simulink model "fan_predictive_maintenance"  (R2024a)
settings: Solver=ode23t  StartTime=0.0  StopTime=30  RelTol=1e-4  AbsTol=1e-4
libraries: fl_lib x13, nesl_utility x5, ee_lib x1, simulink x1
settings Model: Creator=kzlee  LastModifiedBy=kzlee

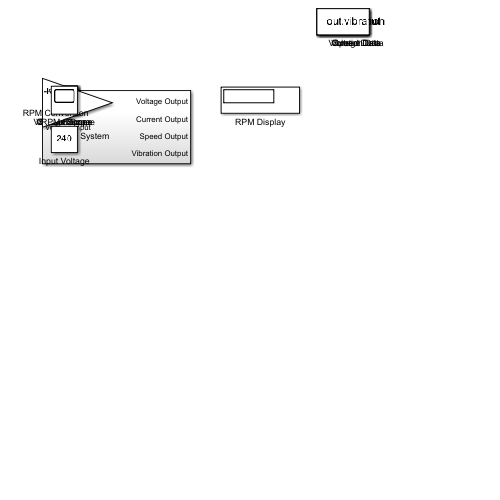
[thumbnail: Simulink's stored preview of the top-level diagram]
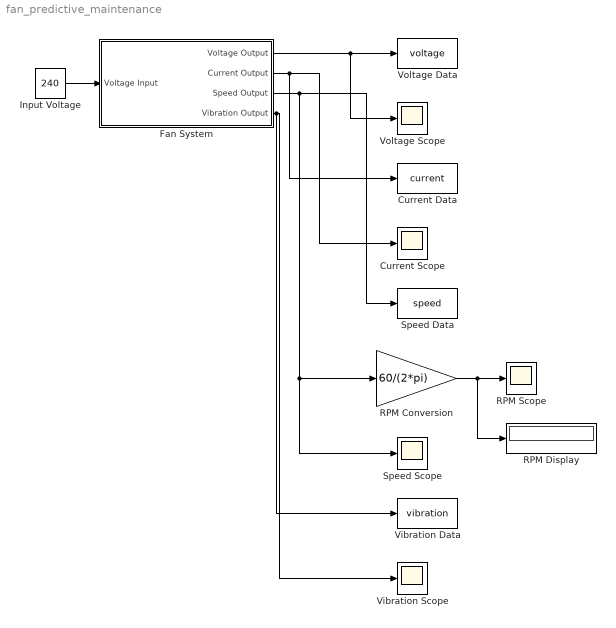
== system fan_predictive_maintenance ==
  Current Data : ToWorkspace  VariableName=current  SaveFormat=Timeseries  SampleTime=-1
  Current Scope : Scope
  Fan System : Subsystem
  Input Voltage : Constant  Value=240
  RPM Conversion : Gain  Gain=60/(2*pi)
  RPM Display : Display
  RPM Scope : Scope
  Speed Data : ToWorkspace  VariableName=speed  SaveFormat=Timeseries  SampleTime=-1
  Speed Scope : Scope
  Vibration Data : ToWorkspace  VariableName=vibration  SaveFormat=Timeseries  SampleTime=-1
  Vibration Scope : Scope
  Voltage Data : ToWorkspace  VariableName=voltage  SaveFormat=Timeseries  SampleTime=-1
  Voltage Scope : Scope
  wires:
  Input Voltage/1 -> Fan System/1(Voltage Input)
  Fan System/3(Speed Output) -> Speed Scope/1, RPM Conversion/1, Speed Data/1
  Fan System/2(Current Output) -> Current Data/1, Current Scope/1
  Fan System/1(Voltage Output) -> Voltage Data/1, Voltage Scope/1
  Fan System/4(Vibration Output) -> Vibration Scope/1, Vibration Data/1
  RPM Conversion/1 -> RPM Display/1, RPM Scope/1

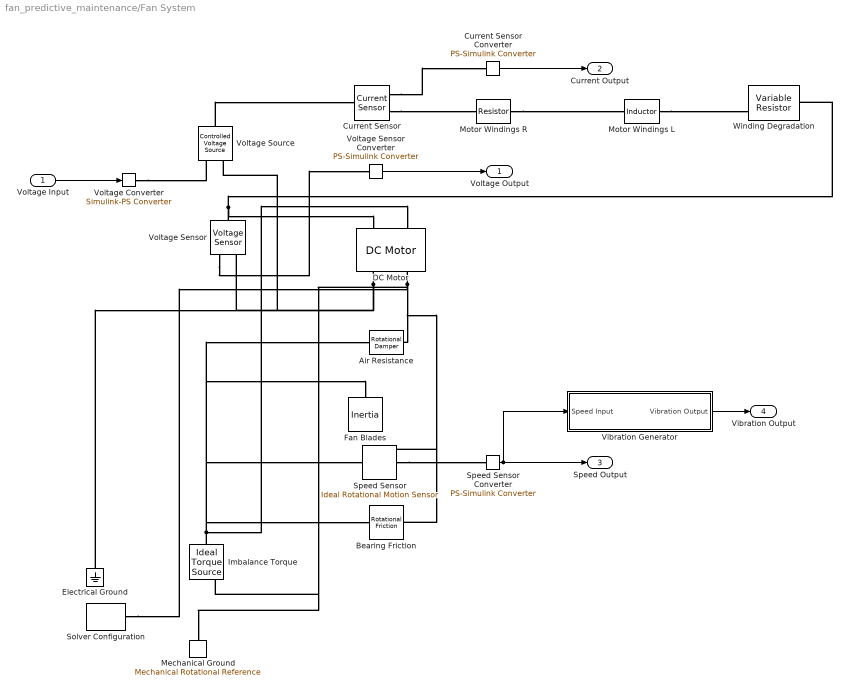
== system fan_predictive_maintenance/Fan System ==
  Voltage Input : Inport
  Air Resistance : fl_lib/Mechanical/Rotational Elements/Rotational Damper  D=0.0045612 N*m*s/rad  w_specify=off  w_priority=None  w=0 rad/s  w_nominal_specify=off  w_nominal_value=1  w_nominal_unit=rad/s  t_specify=off  t_priority=None  t=0 N*m  t_nominal_specify=off  t_nominal_value=1  t_nominal_unit=N*m
  Bearing Friction : fl_lib/Mechanical/Rotational Elements/Rotational Friction  brkwy_trq=25 N*m  brkwy_vel=0.1 rad/s  Col_trq=20 N*m  visc_coef=0.1 N*m*s/rad  w_specify=off  w_priority=None  w=0 rad/s  w_nominal_specify=off  w_nominal_value=1  w_nominal_unit=rad/s  t_specify=off  t_priority=None  t=0 N*m  t_nominal_specify=off  t_nominal_value=1  t_nominal_unit=N*m
  Current Sensor : fl_lib/Electrical/Electrical Sensors/Current Sensor
  Current Sensor Converter : nesl_utility/PS-Simulink Converter  PhysicalDomain=network_engine_domain  SubClassName=ps_output  LeftPortType=input  RightPortType=output  PseudoPeriodic=off  Frequencies=[]  VectorFormat=inherit  Unit=inherit  AffineConversion=off
  DC Motor : ee_lib/Electromechanical/Brushed Motors/DC Motor  field_option=ee.enum.field_option.pm  Rf=100 Ohm  Lf=1 H  Laf=0.15 H  If0=0 A  parameterization=ee.enum.dcparam_option.circuit_param  Ra=1 Ohm  La=0.001 H  emf_or_torque=ee.enum.emf_or_torque.kv  Kv=0.16667 V/rpm  Ki=6.876e-4 N*m/A  T_stall=0.24e-3 N*m  w_max=19100 rpm  w_rated=15000 rpm  P_rated=0.08 W  V_rated=1.5 V  lam_param=ee.enum.lam_param.damping  i_noload=0 A  V_i_noload=1.5 V  J=0.01 cm^2*g  lam=0 N*m*s/rad  speed0=0 rpm  enable_fault_armature=simscape.enum.onoff.off  rev_faulted=1 / 3  G_faulted_armature=1e-5 S  fault_trigger_armature=ee.enum.faults.faultTrigger.temporal  t_fault_armature=1 s  max_permissible_current_armature=inf A  t_fail_on_current_armature=1 s  enable_fault_field=simscape.enum.onoff.off  G_faulted_field=1e-5 S  fault_trigger_field=ee.enum.faults.faultTrigger.temporal  t_fault_field=1 s  max_permissible_current_field=inf A  t_fail_on_current_field=1 s  fault_action=simscape.enum.assert.action.none  alpha=3.93e-3 1/K  Tmeas=25 degC  thermal_mass=100 J/K  initial_temperature=25 degC
  Electrical Ground : fl_lib/Electrical/Electrical Elements/Electrical Reference
  Fan Blades : fl_lib/Mechanical/Rotational Elements/Inertia  inertia=0.001 kg*m^2  num_ports=foundation.enum.numPorts2.one  w_specify=off  w_priority=High  w=0 rad/s  w_nominal_specify=off  w_nominal_value=1  w_nominal_unit=rad/s  t_specify=off  t_priority=None  t=0 N*m  t_nominal_specify=off  t_nominal_value=1  t_nominal_unit=N*m
  Imbalance Torque : fl_lib/Mechanical/Mechanical Sources/Ideal Torque Source
  Mechanical Ground : fl_lib/Mechanical/Rotational Elements/Mechanical Rotational Reference
  Motor Windings L : fl_lib/Electrical/Electrical Elements/Inductor  l=0.001 H  r=0 Ohm  g=1e-9 1/Ohm  i_specify=off  i_priority=None  i=0 A  i_nominal_specify=off  i_nominal_value=1  i_nominal_unit=A  v_specify=off  v_priority=None  v=0 V  v_nominal_specify=off  v_nominal_value=1  v_nominal_unit=V  i_L_specify=off  i_L_priority=High  i_L=0 A  i_L_nominal_specify=off  i_L_nominal_value=1  i_L_nominal_unit=A
  Motor Windings R : fl_lib/Electrical/Electrical Elements/Resistor  R=0.5 Ohm  i_specify=off  i_priority=None  i=0 A  i_nominal_specify=off  i_nominal_value=1  i_nominal_unit=A  v_specify=off  v_priority=None  v=0 V  v_nominal_specify=off  v_nominal_value=1  v_nominal_unit=V
  Solver Configuration : nesl_utility/Solver Configuration  PhysicalDomain=network_engine_domain  SubClassName=solver  LeftPortType=input  RightPortType=generic  Tones=[]  Harmonics=[]  SimulateNoise=off  Profile=off  UseLocalSampling=off  EnableSwitchedLinearOptims=on  FrequencyDomain=off  UseCCode=off  RelTol=0.001  AbsTol=0.001  MinStep=1e-09  ToWorkspace=off  RevertToSquareIcSolve=off  NumHomotopyIterations=100  PhasorMode=off  PhasorModeNumHarmonics=1  ConsistencySolver=NEWTON_XTOL_AFTER_FTOL  IndexReductionMethod=DerivativeReplacement  DoDC=off  ResidualTolerance=1e-09  ConsistencyTolSource=GLOBAL  ConsistencyAbsTol=0.001  ConsistencyRelTol=0.001  ConsistencyTolFactor=0.001  UseLocalSolver=off  LocalSolverChoice=NE_BACKWARD_EULER_ADVANCER  ResolveIndetEquations=on  FunctionEvalNumThread=1  LocalSolverSampleTime=0.001  DoFixedCost=off  MaxNonlinIter=3  MaxModeIter=2  ComputeImpulses=off  ImpulseIterations=2  LinearAlgebra=auto  LinearAlgebraNumThread=0  EquationFormulation=NE_TIME_EF  DelaysMemoryBudget=1024  AutomaticFiltering=on  FilteringTimeConstant=0.001  PartitionStorageMethod=AS_NEEDED  PartitionMemoryBudget=1024  PartitionMethod=ROBUST  MultibodyUseLocalSolver=off  MultibodyLocalSolverChoice=ODE1  MultibodyLocalSolverSampleTime=0.001
  Speed Sensor : fl_lib/Mechanical/Mechanical Sensors/Ideal Rotational Motion Sensor  reference=foundation.enum.MeasurementReference.difference  acceleration_port=false  velocity_port=true  position_port=true  wrap_angle=false  offset=0 rad
  Speed Sensor Converter : nesl_utility/PS-Simulink Converter  PhysicalDomain=network_engine_domain  SubClassName=ps_output  LeftPortType=input  RightPortType=output  PseudoPeriodic=off  Frequencies=[]  VectorFormat=inherit  Unit=inherit  AffineConversion=off
  Vibration Generator : Subsystem
  Voltage Converter : nesl_utility/Simulink-PS Converter  PhysicalDomain=network_engine_domain  SubClassName=ps_input  LeftPortType=input  RightPortType=output  PseudoPeriodic=off  Frequencies=[]  NoiseDistribution=none  NoiseParameters=[]  Unit=1  AffineConversion=off  FilteringAndDerivatives=provide  SimscapeFilterOrder=1  InputFilterTimeConstant=0.001  UdotUserProvided=0
  Voltage Sensor : fl_lib/Electrical/Electrical Sensors/Voltage Sensor
  Voltage Sensor Converter : nesl_utility/PS-Simulink Converter  PhysicalDomain=network_engine_domain  SubClassName=ps_output  LeftPortType=input  RightPortType=output  PseudoPeriodic=off  Frequencies=[]  VectorFormat=inherit  Unit=inherit  AffineConversion=off
  Voltage Source : fl_lib/Electrical/Electrical Sources/Controlled Voltage Source
  Winding Degradation : fl_lib/Electrical/Electrical Elements/Variable Resistor  Rmin=0.1 Ohm  thermalEnable=false  thermal_mass=1 J/K  i_specify=off  i_priority=None  i=0 A  i_nominal_specify=off  i_nominal_value=1  i_nominal_unit=A  v_specify=off  v_priority=None  v=0 V  v_nominal_specify=off  v_nominal_value=1  v_nominal_unit=V  T_specify=off  T_priority=None  T=300 K  T_nominal_specify=off  T_nominal_value=1  T_nominal_unit=K
  Voltage Output : Outport
  Current Output : Outport  Port=2
  Speed Output : Outport  Port=3
  Vibration Output : Outport  Port=4
  wires:
  Voltage Input/1 -> Voltage Converter/1
  Speed Sensor Converter/1 -> Vibration Generator/1(Speed Input), Speed Output/1
  Voltage Sensor Converter/1 -> Voltage Output/1
  Current Sensor Converter/1 -> Current Output/1
  Vibration Generator/1(Vibration Output) -> Vibration Output/1
  connections:
  Voltage Converter/RConn1 -- Voltage Source/RConn1
  Voltage Sensor/LConn1 -- DC Motor/LConn1 -- Winding Degradation/RConn1
  Current Sensor/RConn1 -- Current Sensor Converter/LConn1
  Voltage Sensor/RConn1 -- Voltage Sensor Converter/LConn1
  Current Sensor/RConn2 -- Motor Windings R/LConn1
  Electrical Ground/LConn1 -- Voltage Source/RConn2 -- Voltage Sensor/RConn2 -- DC Motor/RConn1
  Voltage Source/LConn1 -- Current Sensor/LConn1
  Solver Configuration/RConn1 -- Imbalance Torque/RConn2 -- Bearing Friction/RConn1 -- Speed Sensor/RConn1 -- Air Resistance/RConn1 -- Mechanical Ground/LConn1 -- DC Motor/RConn2
  Imbalance Torque/LConn1 -- Air Resistance/LConn1 -- DC Motor/LConn2 -- Speed Sensor/LConn1 -- Bearing Friction/LConn1 -- Fan Blades/LConn1
  Speed Sensor/RConn2 -- Speed Sensor Converter/LConn1
  Motor Windings R/RConn1 -- Motor Windings L/LConn1
  Motor Windings L/RConn1 -- Winding Degradation/LConn2

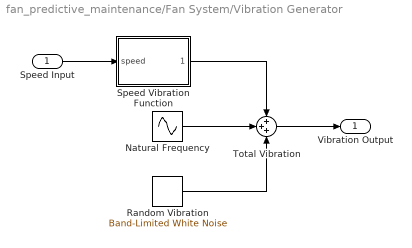
== system fan_predictive_maintenance/Fan System/Vibration Generator ==
  Speed Input : Inport
  Natural Frequency : Sin  Amplitude=0.05  Frequency=50  SampleTime=0
  Random Vibration : simulink/Sources/Band-Limited White Noise  Cov=0.01  Ts=0.1  seed=[23341]
  Speed Vibration Function : MATLAB Function  TreatAsAtomicUnit=on
  Total Vibration : Sum  Inputs=+++
  Vibration Output : Outport
  wires:
  Speed Input/1 -> Speed Vibration Function/1(speed)
  Natural Frequency/1 -> Total Vibration/2
  Speed Vibration Function/1(vibration) -> Total Vibration/1
  Total Vibration/1 -> Vibration Output/1
  Random Vibration/1 -> Total Vibration/3

== matlab function fan_predictive_maintenance/Fan System/Vibration Generator/Speed Vibration Function ==
  settings: updateMethod=DISCRETE  sampleTime=0.001  description=Generate speed-dependent vibration
  data: speed input; vibration output
function vibration = fcn(speed)
    persistent t
    if isempty(t)
        t = 0;
    else
        t = t + 0.01; % Assuming a fixed step size of 0.01s
    end
    freq = speed / (2*pi);
    vibration = 0.1 * sin(2*pi*freq*t);
end
